simulink model "Alapjel_optimalizer"  (R2018b)
settings: Solver=FixedStepAuto  StartTime=0.0  StopTime=4  FixedStep=sampletime  RelTol=1e-3
undefined symbols (not defined in the file or in its folder): Af, alfa, cd, fl, g, k, m, ro, sigbuilder_block
settings Model: Creator=kbene  LastModifiedBy=kbene

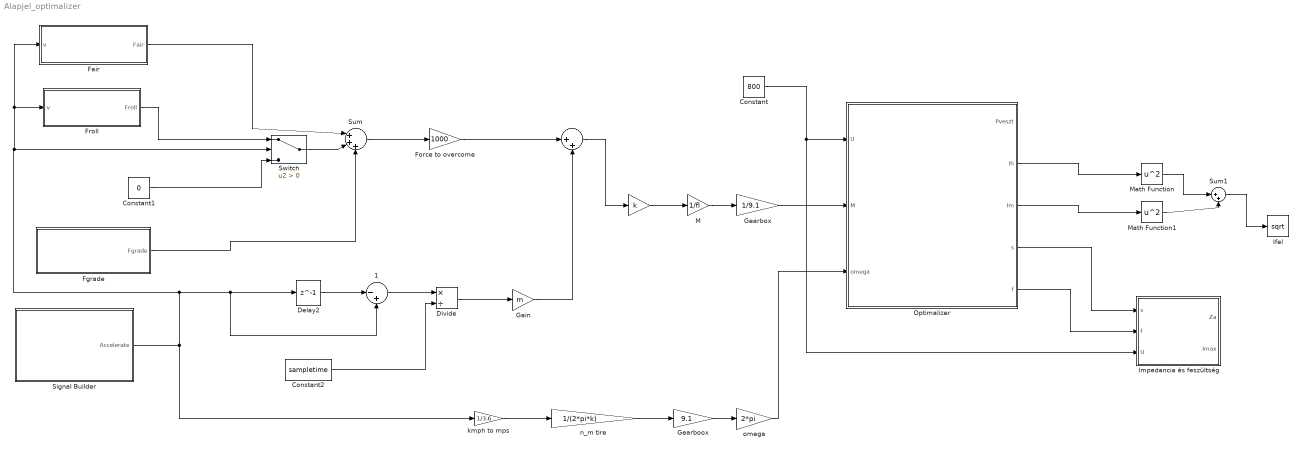
== system Alapjel_optimalizer ==
  " " : Gain  Gain=k
  " " : Sum  Inputs=|++
  " 1" : Sum  Inputs=|-+
  Constant : Constant  Value=800
  Constant1 : Constant  Value=0
  Constant2 : Constant  Value=sampletime
  Delay2 : Delay  DelayLength=1  InitialCondition=0
  Divide : Product  Inputs=*/
  "Fair " : Subsystem
  Fgrade : Subsystem
  Force to overcome : Gain  Gain=1000
  Froll : Subsystem
  Gain : Gain  Gain=m
  "Gearboox " : Gain  Gain=9.1
  "Gearbox " : Gain  Gain=1/9.1
  "Ifel " : Sqrt  SaturateOnIntegerOverflow=on
  "Impedancia és feszültség " : MATLAB Function  TreatAsAtomicUnit=on
  "M " : Gain  Gain=1/fl
  Math Function : Math  Operator=square  SaturateOnIntegerOverflow=on
  Math Function1 : Math  Operator=square  SaturateOnIntegerOverflow=on
  "Optimalizer " : MATLAB Function  TreatAsAtomicUnit=on
  Signal Builder : Subsystem  Tag=STV Subsys  LoadFcn=sigbuilder_block('load');  StartFcn=sigbuilder_block('start');  StopFcn=sigbuilder_block('stop');  ClipboardFcn=sigbuilder_block('clipboard');  mask(Sigbuilder block){tuvar=[0:10]}
      mask help: Simulink:masks:SigbuilderBlock_MD
      mask init:
      | if ~strcmp(get_param(bdroot(gcbh),'SimulationStatus'),'stopped') tuvar = sigbuilder_block('maskInit'); end
      settings: CopyFcn=sigbuilder_block('copy');  DeleteFcn=sigbuilder_block('delete');  ModelCloseFcn=sigbuilder_block('modelClose');  PreSaveFcn=sigbuilder_block('preSave');  PauseFcn=sigbuilder_block('pause');  ContinueFcn=sigbuilder_block('continue');  NameChangeFcn=sigbuilder_block('namechange');  OpenFcn=sigbuilder_block('open',[437.6 199.2 550.4 400 ]);  CloseFcn=sigbuilder_block('close');
      mask Display: plot(0, 0, 100, 100,[2, 2, 32, 32, 2], [68, 8, 8, 68, 68],[32, 2], [38, 38], [32, 19, 2],[53, 60, 44], [32, 17, 17, 2],[16, 16, 31, 31]);txt = getActiveGroup(gcbh);text(2, 100, txt,'verticalAlignment', 'top');
  Sum : Sum  Inputs=|+++
  Sum1 : Sum  Inputs=|++
  Switch : Switch  Criteria=u2 > Threshold
  kmph to mps : Gain  Gain=1/3.6
  "n_m tire " : Gain  Gain=1/(2*pi*k)
  "omega " : Gain  Gain=2*pi
  wires:
  Sum/1 -> Force to overcome/1
  Signal Builder/1(Accelerate) -> Delay2/1, " 1"/2, "Fair "/1(v), Froll/1(v), Switch/2, kmph to mps/1
  Delay2/1 -> " 1"/1
  Constant1/1 -> Switch/3
  Fgrade/1(Fgrade) -> Sum/3
  Constant2/1 -> Divide/2
  " 1"/1 -> Divide/1
  Froll/1(Froll) -> Switch/1
  Force to overcome/1 -> " "/1
  Gain/1 -> " "/2
  " "/1 -> " "/1
  "Fair "/1(Fair) -> Sum/1
  Switch/1 -> Sum/2
  Divide/1 -> Gain/1
  " "/1 -> "M "/1
  "M "/1 -> "Gearbox "/1
  kmph to mps/1 -> "n_m tire "/1
  "n_m tire "/1 -> "Gearboox "/1
  "Gearbox "/1 -> "Optimalizer "/2(M)
  "Gearboox "/1 -> "omega "/1
  "omega "/1 -> "Optimalizer "/3(omega)
  "Optimalizer "/4(s) -> "Impedancia és feszültség "/1(s)
  "Optimalizer "/5(f) -> "Impedancia és feszültség "/2(f)
  Constant/1 -> "Impedancia és feszültség "/3(U), "Optimalizer "/1(U)
  "Optimalizer "/2(Ih) -> Math Function/1
  "Optimalizer "/3(Im) -> Math Function1/1
  Math Function/1 -> Sum1/1
  Math Function1/1 -> Sum1/2
  Sum1/1 -> "Ifel "/1

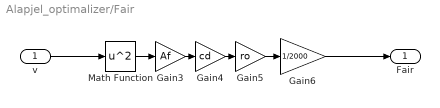
== system Alapjel_optimalizer/Fair  ==
  v : Inport
  Gain3 : Gain  Gain=Af
  Gain4 : Gain  Gain=cd
  Gain5 : Gain  Gain=ro
  Gain6 : Gain  Gain=1/2000
  Math Function : Math  Operator=square  SaturateOnIntegerOverflow=on
  Fair : Outport
  wires:
  Math Function/1 -> Gain3/1
  Gain4/1 -> Gain5/1
  Gain3/1 -> Gain4/1
  Gain5/1 -> Gain6/1
  v/1 -> Math Function/1
  Gain6/1 -> Fair/1

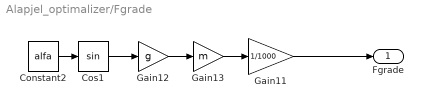
== system Alapjel_optimalizer/Fgrade ==
  Constant2 : Constant  Value=alfa
  Cos1 : Trigonometry
  Gain11 : Gain  Gain=1/1000
  Gain12 : Gain  Gain=g
  Gain13 : Gain  Gain=m
  Fgrade : Outport
  wires:
  Gain13/1 -> Gain11/1
  Constant2/1 -> Cos1/1
  Cos1/1 -> Gain12/1
  Gain12/1 -> Gain13/1
  Gain11/1 -> Fgrade/1

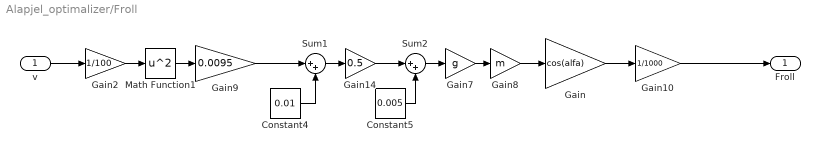
== system Alapjel_optimalizer/Froll ==
  v : Inport
  Constant4 : Constant  Value=0.01
  Constant5 : Constant  Value=0.005
  Gain : Gain  Gain=cos(alfa)
  Gain10 : Gain  Gain=1/1000
  Gain14 : Gain  Gain=0.5
  Gain2 : Gain  Gain=1/100
  Gain7 : Gain  Gain=g
  Gain8 : Gain  Gain=m
  Gain9 : Gain  Gain=0.0095
  Math Function1 : Math  Operator=square  SaturateOnIntegerOverflow=on
  Sum1 : Sum  Inputs=|++
  Sum2 : Sum  Inputs=|++
  Froll : Outport
  wires:
  Gain8/1 -> Gain/1
  Constant4/1 -> Sum1/2
  Sum2/1 -> Gain7/1
  Gain9/1 -> Sum1/1
  Sum1/1 -> Gain14/1
  Gain10/1 -> Froll/1
  Constant5/1 -> Sum2/2
  Math Function1/1 -> Gain9/1
  Gain14/1 -> Sum2/1
  Gain7/1 -> Gain8/1
  Gain2/1 -> Math Function1/1
  v/1 -> Gain2/1
  Gain/1 -> Gain10/1

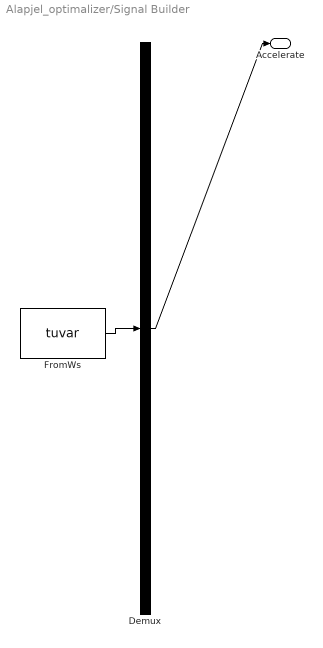
== system Alapjel_optimalizer/Signal Builder ==
  Demux : Demux  Tag=STV Demux  Outputs=1
  FromWs : FromWorkspace  Tag=STV FromWs  VariableName=tuvar  SampleTime=0
      SigBuilderData=|
      | common.afterFinalStr = 'Extrapolate'
      | common.sampleTime = 0
      | dataSet.timeRange = [0 4]
      | dataSet.name = 'Group 1'
      | sbobj.Groups.Name = 'Group 1'
      | sbobj.Groups.Signals.Name = 'Accelerate'
      | sbobj.Groups.Signals.XData = [0 3.3 4]
      | sbobj.Groups.Signals.YData = [0 100 100]
      | sbobj.Groups.TimeRange = [0 4]
  Accelerate : Outport  Tag=STV Outport
  wires:
  FromWs/1 -> Demux/1
  Demux/1 -> Accelerate/1

== matlab function Alapjel_optimalizer/Impedancia és feszültség  ==
  data: s input; f input; Za output; U input; Imax output
function [Za,Imax]=ZU(s, f, U)
Lm=0.0070547
Xm=Lm*2*pi*f
L2=0.0002406
R2=0.0072
X2=L2*2*pi*f
Rm=R2*((1-s)/s)
Z=(((1/(R2+(1i*X2)+Rm))+(1/(1i*Xm)))^(-1))+R2+(1i*X2)
Za=abs(Z)
Imax=abs(U/Z)

== matlab function Alapjel_optimalizer/Optimalizer  ==
  data: U input; Pveszt output; M input; omega input; Ih output; Im output; s output; f output
function [Pveszt,Ih,Im,s,f]=optimal(U,M,omega)
p=1
Lm=0.0070547
R2=0.0072
%Pveszt szamolas, hogy egy megoldas legyen
a=Lm^4
b=-4*(Lm^3)*M*R2
c=((Lm^2)*4*(M^2)*(R2^2))-(8*(Lm^2)*(R2^2)*(M^2))
Pveszt1=((-b)+sqrt((b^2)-(4*a*c)))/(2*a)
Pveszt2=((-b)-sqrt((b^2)-(4*a*c)))/(2*a)
Pveszt=0;
if Pveszt1>0;
    Pveszt=Pveszt1;
elseif Pveszt2>0;
    Pveszt=Pveszt2;
end
a1=2*(Lm^2)*R2
b1=(Lm*2*M*R2)-(Pveszt*(Lm^2))
c1=(M^2)*R2
Ih=sqrt(abs(((-b1)+sqrt(complex((b1^2)-(4*a1*c1))))/(2*a1)))
Im=(M)/(Lm*Ih)
s=(((M*omega)/(3*R2*(Ih^2)))+1)^(-1)
n=(60*omega)/(2*pi)
f=-((n*p)/(60*(s-1)))
